simulink model "gmsk_tx"  (Simulink 7.9)
settings: Solver=FixedStepDiscrete  SolverMode=SingleTasking  StartTime=0.0  StopTime=1e-4  RelTol=1e-3
model workspace (MAT data in the model file):
  Sig = Simulink.Signal
  Sig.DataType = 'auto'
  Sig.Dimensions = -1
  Sig.DimensionsMode = 'auto'
  Sig.Complexity = 'auto'
  Sig.SampleTime = -1
  Sig.SamplingMode = 'auto'
  sin_lut_length = Simulink.Parameter
  sin_lut_length.Value = 64
  sin_lut_length.DataType = 'auto'
  Sig1 = Simulink.Signal
  Sig1.DataType = 'auto'
  Sig1.Dimensions = -1
  Sig1.DimensionsMode = 'auto'
  Sig1.Complexity = 'auto'
  Sig1.SampleTime = -1
  Sig1.SamplingMode = 'auto'
PreLoadFcn:
  | gmsk_syn_init;
undefined symbols (not defined in the file): gaussfir, gmsk_syn_params
libraries: shlslibv1 x17, dspsigops x3, commrandsrc2 x1, commdigbbndcpm2 x1, commutil2 x1
settings Model: synDspstartup=OK  Creator=sszilvasi  LastModifiedBy=sszilvasi
settings DataIOCC: SaveOutput=off  SignalLogging=off  SaveTime=off
settings OptimizationCC: InlineParams=on
settings DebuggingCC: AlgebraicLoopMsg=error  InheritedTsInSrcMsg=none

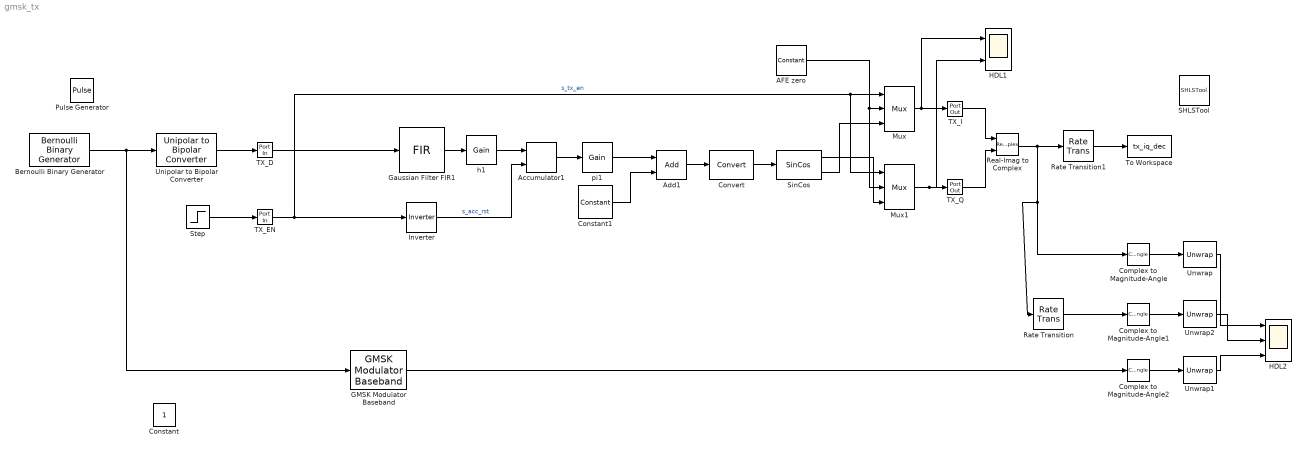
== system gmsk_tx ==
  AFE zero : shlslibv1/Sources/Constant  syn_cst_val=0  syn_cst_fl=9  syn_cst_dt=signed  syn_cst_rnd=on  syn_cst_st=-1  synBlockType=primitive  synLatency=0  synBlockId=15
  Accumulator1 : shlslibv1/Math Functions/Accumulator  syn_acc_opr=+=  syn_out_f=Automatic  syn_out_wl=16  syn_out_fl=5  syn_out_dt=signed  syn_rst_port=on  syn_en_port=off  syn_ovf_port=off  synBlockType=primitive  synLatency=0  synBlockId=105
  Add1 : shlslibv1/Math Functions/Add  syn_add_opr=++  syn_out_f=Automatic  syn_out_wl=5  syn_out_fl=5  syn_out_dt=unsigned  syn_out_sat=off  syn_out_rnd=Floor (Truncate)  synBlockType=primitive  synLatency=0  synBlockId=96  syn_sum_of_rows=off
  Bernoulli Binary Generator : commrandsrc2/Bernoulli Binary Generator  P=0.5  seed=61  Ts=gmsk_syn_params.Ts*gmsk_syn_params.symbol_time  frameBased=off  sampPerFrame=1  orient=off  outDataType=double
  Complex to Magnitude-Angle : ComplexToMagnitudeAngle  Output=Angle
  Complex to Magnitude-Angle1 : ComplexToMagnitudeAngle  Output=Angle
  Complex to Magnitude-Angle2 : ComplexToMagnitudeAngle  Output=Angle
  Constant : Constant  SampleTime=gmsk_syn_params.Ts*gmsk_syn_params.symbol_time
  Constant1 : shlslibv1/Sources/Constant  syn_cst_val=.5  syn_cst_fl=1  syn_cst_dt=signed  syn_cst_rnd=on  syn_cst_st=-1  synBlockType=primitive  synLatency=0  synBlockId=15
  Convert : shlslibv1/Signal Operations/Convert  syn_preshift_opr=none  syn_preshift_bits=0  syn_preshift_val=0  syn_out_f=Specify  syn_out_wl=11  syn_out_fl=8  syn_out_dt_sync=signed  syn_out_sat=off  syn_out_rnd=Floor (Truncate)  syn_inh_port=off  syn_inh_st=off  syn_inh_stf=1  synBlockType=primitive  synLatency=0  synBlockId=4
  GMSK Modulator Baseband : commdigbbndcpm2/GMSK Modulator Baseband  inputType=Bit  BT=.5  pulseLength=2  preHistory=1  phaseOffset=0  samplesPerSymbol=gmsk_syn_params.gauss_oversampling  RateOptions=Allow multirate processing  outDataType=double
  Gaussian Filter FIR1 : shlslibv1/Filtering/FIR  syn_coef_vec=gaussfir(0.5,1,gmsk_syn_params.gauss_oversampling)  syn_coef_fl=15  syn_coef_rnd=Nearest  syn_show_q=off  syn_dp_f=Automatic  syn_dp_wl=16  syn_dp_fl=8  syn_dp_sat=off  syn_dp_rnd=Floor (Truncate)  syn_out_f=Full Precision  syn_out_wl=16  syn_out_fl=8  syn_out_dt=signed  syn_out_sat=off  syn_out_rnd=Floor (Truncate)  syn_rst_port=off  syn_en_port=off  synBlockType=primitive  synLatency=0  synBlockId=80
  HDL1 : Scope  NumInputPorts=2
      settings: YMin=-5~-5  YMax=5~5
  HDL2 : Scope  NumInputPorts=3
      settings: TimeRange=0.0002999999999999999  YMin=775~750~-52.5  YMax=1125~1450~-5  SaveName=ScopeData4
  Inverter : shlslibv1/Math Functions/Inverter  syn_out_f=Automatic  syn_out_wl=16  syn_out_fl=8  syn_out_dt=signed  synBlockType=primitive  synLatency=0  synBlockId=10
  Mux : shlslibv1/Signal Operations/Mux  syn_in_nb=2  syn_out_f=Full Precision  syn_out_wl=16  syn_out_fl=8  syn_out_dt=signed  synBlockType=primitive  synLatency=0  synBlockId=16
  Mux1 : shlslibv1/Signal Operations/Mux  syn_in_nb=2  syn_out_f=Full Precision  syn_out_wl=16  syn_out_fl=8  syn_out_dt=signed  synBlockType=primitive  synLatency=0  synBlockId=16
  Pulse Generator : DiscretePulseGenerator  Period=gmsk_syn_params.symbol_time*8  PulseWidth=gmsk_syn_params.symbol_time  PhaseDelay=gmsk_syn_params.symbol_time*1  SampleTime=gmsk_syn_params.Ts
  Rate Transition : RateTransition  OutPortSampleTime=gmsk_syn_params.Ts*gmsk_syn_params.symbol_time/gmsk_syn_params.gauss_oversampling
  Rate Transition1 : RateTransition  OutPortSampleTime=gmsk_syn_params.Ts
  Real-Imag to Complex : RealImagToComplex
  SHLSTool : shlslibv1/SHLSTool  synBlockType=tool  syn_dsp_mode=FPGA
  SinCos : shlslibv1/Math Functions/SinCos  syn_sincos_opr=sin&cos  syn_sincos_amp=1  syn_out_f=Specify  syn_out_wl=10  syn_out_fl=8  synBlockType=primitive  synLatency=1  synBlockId=65
  Step : Step  Time=gmsk_syn_params.Ts*100  SampleTime=gmsk_syn_params.Ts
  TX_D : shlslibv1/Ports & Subsystems/Port In  syn_out_wl=16  syn_out_fl=14  syn_out_dt=signed  syn_out_st=gmsk_syn_params.Ts  syn_capture=on  syn_register=off  syn_out_sat=on  syn_out_rnd=on  synBlockType=port  synLatency=0  synBlockId=0
  TX_EN : shlslibv1/Ports & Subsystems/Port In  syn_out_wl=1  syn_out_fl=0  syn_out_dt=unsigned  syn_out_st=gmsk_syn_params.Ts  syn_capture=on  syn_register=off  syn_out_sat=off  syn_out_rnd=on  synBlockType=port  synLatency=0  synBlockId=0
  TX_I : shlslibv1/Ports & Subsystems/Port Out  syn_capture=on  syn_register=off  synBlockType=port  synLatency=0  synBlockId=1
  TX_Q : shlslibv1/Ports & Subsystems/Port Out  syn_capture=on  syn_register=off  synBlockType=port  synLatency=0  synBlockId=1
  To Workspace : ToWorkspace  VariableName=tx_iq_dec  SampleTime=-1  SaveFormat=Timeseries
  Unipolar to Bipolar Converter : commutil2/Unipolar to Bipolar Converter  M=2  polarity=Positive  dataType=Inherit via internal rule
  Unwrap : dspsigops/Unwrap  tol=pi  InputProcessing=Columns as channels (frame based)  running=off
  Unwrap1 : dspsigops/Unwrap  tol=pi  InputProcessing=Columns as channels (frame based)  running=off
  Unwrap2 : dspsigops/Unwrap  tol=pi  InputProcessing=Columns as channels (frame based)  running=off
  h1 : shlslibv1/Math Functions/Gain  syn_gain_val=1/gmsk_syn_params.gauss_oversampling  syn_gain_fl=15  syn_gain_dt=signed  syn_gain_rnd=on  syn_out_f=Full Precision  syn_out_wl=16  syn_out_fl=8  syn_out_dt=signed  syn_out_sat=off  syn_out_rnd=Floor (Truncate)  synBlockType=primitive  synLatency=0  synBlockId=3  syn_opr_mode=0
  pi1 : shlslibv1/Math Functions/Gain  syn_gain_val=1/4  syn_gain_fl=15  syn_gain_dt=signed  syn_gain_rnd=on  syn_out_f=Full Precision  syn_out_wl=16  syn_out_fl=8  syn_out_dt=signed  syn_out_sat=off  syn_out_rnd=Floor (Truncate)  synBlockType=primitive  synLatency=0  synBlockId=3  syn_opr_mode=0
  wires:
  TX_I/1 -> Real-Imag to Complex/1
  TX_Q/1 -> Real-Imag to Complex/2
  Real-Imag to Complex/1 -> Complex to Magnitude-Angle/1, Rate Transition/1, Rate Transition1/1
  TX_D/1 -> Gaussian Filter FIR1/1
  Step/1 -> TX_EN/1
  Unipolar to Bipolar Converter/1 -> TX_D/1
  GMSK Modulator Baseband/1 -> Complex to Magnitude-Angle2/1
  Complex to Magnitude-Angle/1 -> Unwrap/1
  Complex to Magnitude-Angle2/1 -> Unwrap1/1
  Unwrap/1 -> HDL2/1
  Bernoulli Binary Generator/1 -> Unipolar to Bipolar Converter/1, GMSK Modulator Baseband/1
  Add1/1 -> Convert/1
  pi1/1 -> Add1/1
  Constant1/1 -> Add1/2
  Accumulator1/1 -> pi1/1
  h1/1 -> Accumulator1/1
  Gaussian Filter FIR1/1 -> h1/1
  TX_EN/1 -> Mux/1, Mux1/1, Inverter/1  "s_tx_en"
  Unwrap1/1 -> HDL2/3
  Complex to Magnitude-Angle1/1 -> Unwrap2/1
  Rate Transition/1 -> Complex to Magnitude-Angle1/1
  Unwrap2/1 -> HDL2/2
  Rate Transition1/1 -> To Workspace/1
  AFE zero/1 -> Mux/2, Mux1/2
  Mux/1 -> TX_I/1, HDL1/1
  Mux1/1 -> TX_Q/1, HDL1/2
  SinCos/2 -> Mux/3
  SinCos/1 -> Mux1/3
  Inverter/1 -> Accumulator1/2  "s_acc_rst"
  Convert/1 -> SinCos/1
